simulink model "sfcndemo_runtime"  (Simulink 7.6)
settings: Solver=FixedStepDiscrete  StartTime=0.0  StopTime=inf  RelTol=1e-3
PreLoadFcn:
  | gainVal=5;gainVal2=int8(5);
Description:
  | Run-Time Parameter C-MEX S-functions with Real-Time Workshop details
settings Model: Creator=The MathWorks Inc.  CovMetricSettings=d  ExtModeAutoUpdateStatusClock=off  TunableVars=gainVal,gainVal2  TunableVarsStorageClass=Auto,Auto  TunableVarsTypeQualifier=,
settings DataIOCC: SignalLoggingName=sigsOut
settings OptimizationCC: BlockReduction=off  BooleanDataType=off  InlineParams=on  InlineInvariantSignals=on  InitFltsAndDblsToZero=on
settings DebuggingCC: SaveWithParameterizedLinksMsg=none  SignalResolutionControl=TryResolveAllWithWarning  SolverPrmCheckMsg=none  MultiTaskDSMMsg=warning  MultiTaskCondExecSysMsg=none
settings HardwareCC: ProdHWDeviceType=Specified  TargetUnknown=on
settings RTWCC: RetainRTWFile=on  IncludeERTFirstTime=on
settings CodeAppCC: CustomSymbolStrFcn=$F$N$M
settings GRTTargetCC: TargetFcnLib=ansi_tfl_tmw.mat

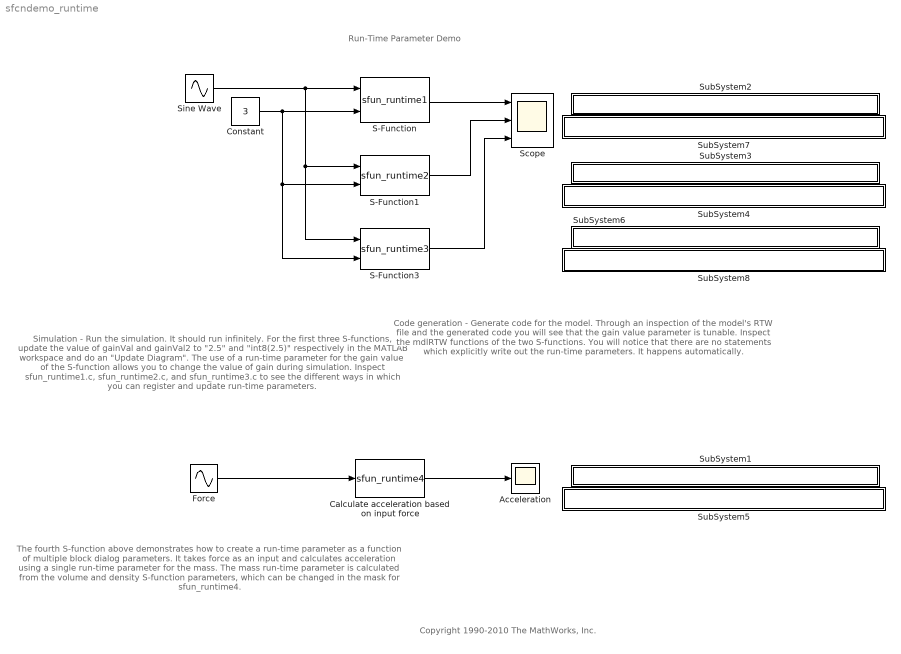
== system sfcndemo_runtime ==
  note: Run-Time Parameter Demo
  note: Simulation -
      | Run the simulation. It should run infinitely.
      | For the first three S-functions, update the value of gainVal and
      | gainVal2 to "2.5" and "int8(2.5)" respectively in the MATLAB
      | workspace and do an "Update Diagram". The use of a run-time
      | parameter for the gain value of the S-function allows you to
      | change the value of gain during simulation.
      |
      | Inspect sfun_runtime1.c, sfun_runtime2.c, and sfun_runtime3.c
      | to see the different ways in which you can register and update
      | run-time parameters.
  note: Code generation -
      | Generate code for the model. Through an inspection of the
      | model's RTW file and the generated code you will see that the
      | gain value parameter is tunable.
      |
      | Inspect the mdlRTW functions of the two S-functions. You will
      | notice that there are no statements which explicitly write out the
      | run-time parameters. It happens automatically.
  note: Copyright 1990-2010 The MathWorks, Inc.
  note: The fourth S-function above demonstrates how to create a
      | run-time parameter as a function of multiple block dialog parameters.
      | It takes force as an input and calculates acceleration using a single
      | run-time parameter for the mass. The mass run-time parameter is
      | calculated from the volume and density S-function parameters,
      | which can be changed in the mask for sfun_runtime4.
  Acceleration : Scope
      settings: YMin=-1  YMax=1
  Calculate acceleration based on input force : S-Function  FunctionName=sfun_runtime4  Parameters=vol,den  EnableBusSupport=off  mask{vol=2, den=5}
      mask prompts: vol "Volume:"; den "Density:"
      mask help:
      | S-function demonstration using one run-time parameter calculated
      | from two S-function dialog parameters.
      |
      | The S-function calculates the acceleration of a body defined by
      | volume and density given an input force.
      |
      | Mass is stored in a run-time parameter.
      |
      | Mass = Volume * Density
      | Acceleration = Force / Mass
  Constant : Constant  Value=3
  Force : Sin  Amplitude=10  SampleTime=0
  S-Function : S-Function  FunctionName=sfun_runtime1  Parameters='++',gainVal,'SumTimesGain'  EnableBusSupport=off
  S-Function1 : S-Function  FunctionName=sfun_runtime2  Parameters='++',gainVal,'SumTimesGain'  EnableBusSupport=off
  S-Function3 : S-Function  FunctionName=sfun_runtime3  Parameters='++',gainVal2,'SumTimesGain'  EnableBusSupport=off
  Scope : Scope  NumInputPorts=3
      settings: TimeRange=4  YMin=5~5~5  YMax=20~20~20
  Sine Wave : Sin  SampleTime=0.1
  SubSystem1 : Subsystem  mask{filename=sfun_runtime4.c}
      mask init:
      | x=sfundemo_maskdisp;
      settings: AttributesFormatString=\n  OpenFcn=sfundemo_openfcn
      mask Display: disp(x);
  SubSystem2 : Subsystem  mask{filename=sfun_runtime1.c}
      mask init:
      | x=sfundemo_maskdisp;
      settings: AttributesFormatString=\n  OpenFcn=sfundemo_openfcn
      mask Display: disp(x);
  SubSystem3 : Subsystem  mask{filename=sfun_runtime2.c}
      mask init:
      | x=sfundemo_maskdisp;
      settings: AttributesFormatString=\n  OpenFcn=sfundemo_openfcn
      mask Display: disp(x);
  SubSystem4 : Subsystem  mask{filename=sfun_runtime2.tlc}
      mask init:
      | x=sfundemo_maskdisp;
      settings: AttributesFormatString=\n  OpenFcn=sfundemo_openfcn
      mask Display: disp(x);
  SubSystem5 : Subsystem  mask{filename=sfun_runtime4.tlc}
      mask init:
      | x=sfundemo_maskdisp;
      settings: AttributesFormatString=\n  OpenFcn=sfundemo_openfcn
      mask Display: disp(x);
  SubSystem6 : Subsystem  mask{filename=sfun_runtime3.c}
      mask init:
      | x=sfundemo_maskdisp;
      settings: AttributesFormatString=\n  OpenFcn=sfundemo_openfcn
      mask Display: disp(x);
  SubSystem7 : Subsystem  mask{filename=sfun_runtime1.tlc}
      mask init:
      | x=sfundemo_maskdisp;
      settings: AttributesFormatString=\n  OpenFcn=sfundemo_openfcn
      mask Display: disp(x);
  SubSystem8 : Subsystem  mask{filename=sfun_runtime3.tlc}
      mask init:
      | x=sfundemo_maskdisp;
      settings: AttributesFormatString=\n  OpenFcn=sfundemo_openfcn
      mask Display: disp(x);
  wires:
  Sine Wave/1 -> S-Function/1, S-Function1/1, S-Function3/1
  Constant/1 -> S-Function/2, S-Function1/2, S-Function3/2
  S-Function/1 -> Scope/1
  S-Function1/1 -> Scope/2
  S-Function3/1 -> Scope/3
  Calculate acceleration based on input force/1 -> Acceleration/1
  Force/1 -> Calculate acceleration based on input force/1

== system sfcndemo_runtime/SubSystem1 ==

== system sfcndemo_runtime/SubSystem2 ==

== system sfcndemo_runtime/SubSystem3 ==

== system sfcndemo_runtime/SubSystem4 ==

== system sfcndemo_runtime/SubSystem5 ==

== system sfcndemo_runtime/SubSystem6 ==

== system sfcndemo_runtime/SubSystem7 ==

== system sfcndemo_runtime/SubSystem8 ==
